simulink model "Transform_image_geometry"  (Simulink 10.1)
settings: Solver=VariableStepAuto  StartTime=0.0  StopTime=10.0  RelTol=1e-3
libraries: visionsources x1
settings Model: Creator=lacak  LastModifiedBy=lacak
settings DataIOCC: SaveFormat=Dataset  ReturnWorkspaceOutputs=on
settings OptimizationCC: LifeSpan=auto
settings DebuggingCC: UnderspecifiedInitializationDetection=Simplified  MergeDetectMultiDrivingBlocksExec=error  SFUnexpectedBacktrackingDiag=error  SFNoUnconditionalDefaultTransitionDiag=error  SFExecutionAtInitializationDiag=warning  ArithmeticOperatorsInVariantConditions=error
settings HardwareCC: ProdBitPerPointer=64  ProdBitPerSizeT=64  ProdBitPerPtrDiffT=64  ProdLargestAtomicFloat=Float  ProdIntDivRoundTo=Zero  ProdEndianess=LittleEndian  ProdWordSize=64  ProdHWDeviceType=Intel->x86-64 (Windows64)
settings ModelReferenceCC: PropagateSignalLabelsOutOfModel=on
settings SFSimCC: SimUseLocalCustomCode=on  CustomCodeUndefinedFunction=FilterOut
settings RTWCC: RTWUseLocalCustomCode=on
settings CodeAppCC: StateflowObjectComments=off
settings GRTTargetCC: TargetLangStandard=C99 (ISO)  CombineOutputUpdateFcns=on  GRTInterface=off
settings ConfigComp: CovMetricSettings=dwe  CovHtmlReporting=off  CovSaveCumulativeToWorkspaceVar=off  CovSaveSingleToWorkspaceVar=off  CovExternalEMLEnable=on

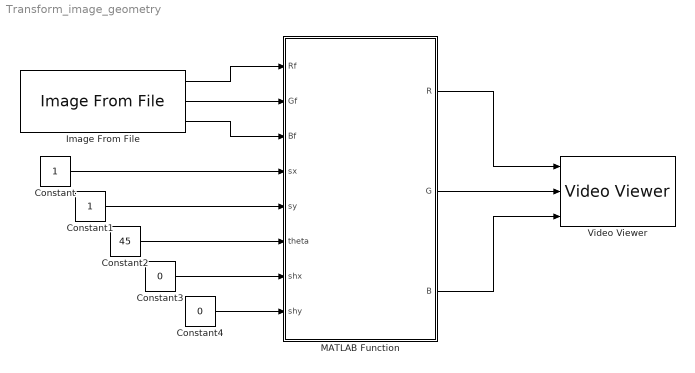
== system Transform_image_geometry ==
  Constant : Constant
  Constant1 : Constant
  Constant2 : Constant  Value=45
  Constant3 : Constant  Value=0
  Constant4 : Constant  Value=0
  Image From File : visionsources/Image From File  Tag=vipblks_nd  FileName=testImg.jpg  Ts=inf  imagePorts=Separate color signals  OutPortLabels=R|G|B  ImageDataType=Inherit from input image  sdImageDataType=uint(8)  Signed=on  WordLength=16  FractionLengthMode=User-defined  FractionLength=15
  MATLAB Function : MATLAB Function  TreatAsAtomicUnit=on
  Video Viewer : VideoViewer  imagePorts=separate color signals  FigPos=[1 822 1536 724]
  wires:
  Constant4/1 -> MATLAB Function/8(shy)
  Constant3/1 -> MATLAB Function/7(shx)
  Constant2/1 -> MATLAB Function/6(theta)
  Constant1/1 -> MATLAB Function/5(sy)
  Constant/1 -> MATLAB Function/4(sx)
  MATLAB Function/1(R) -> Video Viewer/1
  MATLAB Function/2(G) -> Video Viewer/2
  MATLAB Function/3(B) -> Video Viewer/3
  Image From File/1 -> MATLAB Function/1(Rf)
  Image From File/2 -> MATLAB Function/2(Gf)
  Image From File/3 -> MATLAB Function/3(Bf)

== matlab function MATLAB Function ==
  data: Rf input double; R output double; Gf input double; Bf input double; sx input double; sy input double; theta input double; shx input double; shy input double; G output double; B output double
function [R, G, B] = fcn(Rf, Gf, Bf, sx, sy, theta, shx, shy)

tx=0; ty=0;

shear = eye(3,3);
shear(1,2) = shx;
shear(2,1) = shy;

scale = eye(3,3);
scale(1,1) = sx;
scale(2,2) = sy;

tplus = eye(3,3);
tminus = eye(3,3);
rotation = eye(3,3);
xc = floor(size(Rf, 1) / 2);
yc = floor(size(Rf, 2) / 2);

tplus(1,3) = xc;
tplus(2,3) = yc;
rotation(1,1) = cos(theta * pi / 180);
rotation(1,2) = -1 * sin(theta * pi / 180);
rotation(2,1) = sin(theta * pi / 180);
rotation(2,2) = cos(theta * pi / 180);

translate = eye(3,3);
translate(1,3) = tx;
translate(2,3) = ty;

R = zeros(size(Rf,1), size(Rf,2));
G = zeros(size(Rf,1), size(Rf,2));
B = zeros(size(Rf,1), size(Rf,2));

T = shear * scale * tplus * rotation * tminus * translate;

for u=1:size(Rf,1)
    for v=1:size(Rf,2)
        uv = [u;v;1];
        xy = floor(T*uv);
        x=xy(1); y=xy(2);
        if x>0 && y>0 && x<size(Rf,1) && y<size(Rf,2)
            R(u,v) = Rf(x,y);
            G(u,v) = Gf(x,y);
            B(u,v) = Bf(x,y);
        end
    end
end

end
